simulink model "Magnetorquer"  (R2023b)
settings: Solver=FixedStepAuto  StartTime=0.0  StopTime=30  FixedStep=0.005  MaxStep=0.05  RelTol=1e-3
model workspace (MAT data in the model file):
  A = Simulink.Parameter
  A.Value = 0.00020106192
  A.DataType = 'auto'
  A.Complexity = 'real'
  A.Dimensions = [1 1]
  L = Simulink.Parameter
  L.Value = 0.1
  L.DataType = 'auto'
  L.Complexity = 'real'
  L.Dimensions = [1 1]
  M_s = Simulink.Parameter
  M_s.Value = 1600000
  M_s.DataType = 'auto'
  M_s.Complexity = 'real'
  M_s.Dimensions = [1 1]
  R = Simulink.Parameter
  R.Value = 4.0416
  R.DataType = 'auto'
  R.Complexity = 'real'
  R.Dimensions = [1 1]
  Sig = Simulink.Signal
  Sig.DataType = 'auto'
  Sig.Dimensions = -1
  Sig.DimensionsMode = 'auto'
  Sig.Complexity = 'auto'
  Sig.SampleTime = -1
  Sig.SamplingMode = 'auto'
  a = Simulink.Parameter
  a.Value = 1100
  a.DataType = 'auto'
  a.Complexity = 'real'
  a.Dimensions = [1 1]
  alpha = Simulink.Parameter
  alpha.Value = 0.0016
  alpha.DataType = 'auto'
  alpha.Complexity = 'real'
  alpha.Dimensions = [1 1]
  c = Simulink.Parameter
  c.Value = 0.2
  c.DataType = 'auto'
  c.Complexity = 'real'
  c.Dimensions = [1 1]
  k = Simulink.Parameter
  k.Value = 400
  k.DataType = 'auto'
  k.Complexity = 'real'
  k.Dimensions = [1 1]
  mu_0 = Simulink.Parameter
  mu_0.Value = 1.25663706212e-06
  mu_0.DataType = 'auto'
  mu_0.Complexity = 'real'
  mu_0.Dimensions = [1 1]
  n = Simulink.Parameter
  n.Value = 1000
  n.DataType = 'auto'
  n.Complexity = 'real'
  n.Dimensions = [1 1]
values from neighbouring files (symbols this model uses):
  a = 15    [quaternionTest.m]
  R = [1 - 2*(qj^2 + qk^2),  2*(qi*qj - qk*qr),   2*(qi*qk + qj*qr) ... (first row only)    [quat2rotmat.m]
settings Model: SnapshotBufferSize=20  SnapshotInterval=1  Creator=andrea  LastModifiedBy=andrea
settings SolverCC: ZeroCrossAlgorithm=Adaptive  SolverResetMethod=Robust
settings HardwareCC: ProdBitPerLong=64  ProdHWDeviceType=Intel->x86-64 (Linux 64)

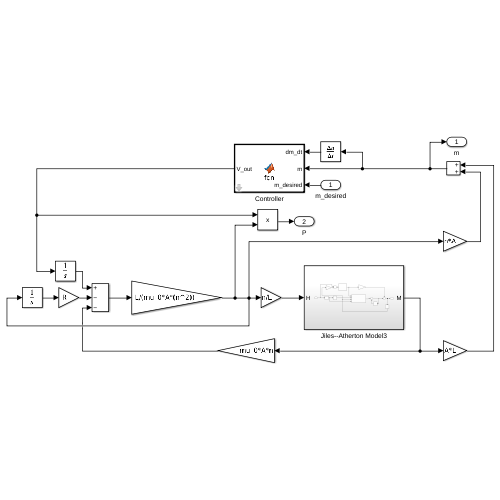
[thumbnail: Simulink's stored preview of the top-level diagram]
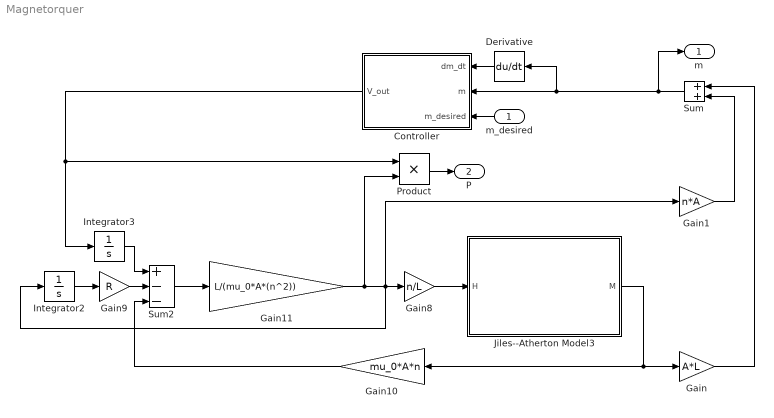
== system Magnetorquer ==
  m_desired : Inport
  Controller : MATLAB Function  TreatAsAtomicUnit=on  SystemSampleTime=0.005  mask{V=3.3, dt=0.005, e=0.5}
  Derivative : Derivative
  Gain : Gain  Gain=A*L
  Gain1 : Gain  Gain=n*A
  Gain10 : Gain  Gain=mu_0*A*n
  Gain11 : Gain  Gain=L/(mu_0*A*(n^2))
  Gain8 : Gain  Gain=n/L
  Gain9 : Gain  Gain=R
  Integrator2 : Integrator
  Integrator3 : Integrator
  Jiles--Atherton Model3 : Subsystem
  Product : Product
  Sum : Sum
  Sum2 : Sum  Inputs=+--
  m : Outport
  P : Outport  Port=2
  wires:
  Gain8/1 -> Jiles--Atherton Model3/1(H)
  Integrator2/1 -> Gain9/1
  Gain9/1 -> Sum2/2
  Integrator3/1 -> Sum2/1
  Sum2/1 -> Gain11/1
  Gain1/1 -> Sum/2
  Gain/1 -> Sum/1
  Sum/1 -> m/1, Derivative/1, Controller/2(m)
  Derivative/1 -> Controller/1(dm_dt)
  Gain11/1 -> Product/2, Gain1/1, Integrator2/1, Gain8/1
  Gain10/1 -> Sum2/3
  Jiles--Atherton Model3/1(M) -> Gain/1, Gain10/1
  Controller/1(V_out) -> Integrator3/1, Product/1
  m_desired/1 -> Controller/3(m_desired)
  Product/1 -> P/1

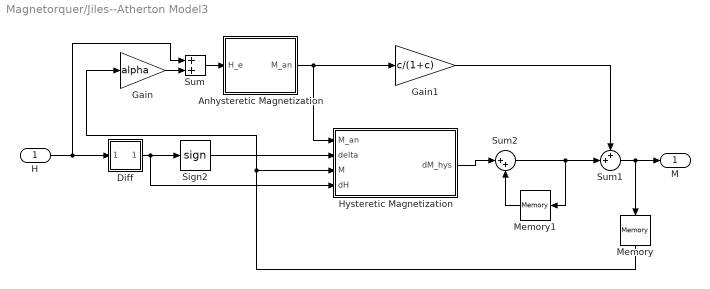
== system Magnetorquer/Jiles--Atherton Model3 ==
  H : Inport
  Anhysteretic Magnetization : MATLAB Function  TreatAsAtomicUnit=on  mask{M_s=M_s, a=a}
  Diff : Subsystem
  Gain : Gain  Gain=alpha
  Gain1 : Gain  Gain=c/(1+c)
  Hysteretic Magnetization : MATLAB Function  TreatAsAtomicUnit=on  mask{c=c, alpha=alpha, k=k}
  Memory : Memory
  Memory1 : Memory
  Sign2 : Signum
  Sum : Sum
  Sum1 : Sum  Inputs=++|
  Sum2 : Sum  Inputs=|++
  M : Outport
  wires:
  H/1 -> Sum/1, Diff/1(In1)
  Diff/1(Out1) -> Hysteretic Magnetization/4(dH), Sign2/1
  Sign2/1 -> Hysteretic Magnetization/2(delta)
  Gain/1 -> Sum/2
  Sum/1 -> Anhysteretic Magnetization/1(H_e)
  Memory/1 -> Hysteretic Magnetization/3(M), Gain/1
  Anhysteretic Magnetization/1(M_an) -> Gain1/1, Hysteretic Magnetization/1(M_an)
  Sum1/1 -> Memory/1, M/1
  Sum2/1 -> Memory1/1, Sum1/2
  Memory1/1 -> Sum2/2
  Hysteretic Magnetization/1(dM_hys) -> Sum2/1
  Gain1/1 -> Sum1/1

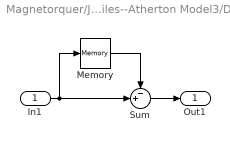
== system Magnetorquer/Jiles--Atherton Model3/Diff ==
  In1 : Inport
  Memory : Memory
  Sum : Sum  Inputs=-+|
  Out1 : Outport
  wires:
  In1/1 -> Memory/1, Sum/2
  Memory/1 -> Sum/1
  Sum/1 -> Out1/1

== matlab function Magnetorquer/Controller ==
  data: V_out output; dm_dt input; m input; m_desired input; V parameter; e parameter; dt parameter
function V_out = fcn(dm_dt, m, m_desired, V, e, dt)

if abs(m_desired-m) < e
    V_out = 0;
elseif abs((m_desired + dm_dt*dt)-m) < e
    V_out = 0;
else
    V_out = V*sign(m_desired-m);
end

== matlab function Magnetorquer/Jiles--Atherton Model3/Anhysteretic Magnetization ==
  data: H_e input; M_an output; M_s parameter; a parameter
function M_an = fcn(H_e, M_s, a)

if abs(H_e/a) <= 1e-5
    M_an = (1/3)*H_e/a;
else
    M_an = M_s * (coth(H_e/a)-a/H_e);
end

%H_e
%M_an

== matlab function Magnetorquer/Jiles--Atherton Model3/Hysteretic Magnetization ==
  data: M_an input; delta input; M input; dH input; dM_hys output; c parameter; k parameter; alpha parameter
function dM_hys = fcn(M_an, delta, M, dH, c, k, alpha)

if (M_an-M>0) && (delta<0)
    delta_m = 0;
elseif (M_an-M<0) && (delta>0)
    delta_m = 0;
else
    delta_m = 1;
end

if delta == 0
    delta = 1;
end

%dH
%dM_an
%delta
%M
%alpha
%thing1=(delta_m/(1+c))
%thing2=((M_an-M)/(delta*k-alpha*(M_an-M)))
%thing3=(M_an-M)
%thing4=(delta*k-alpha*(M_an-M))
%delta
dM_hys = (delta_m/(1+c))*((M_an-M)/(delta*k-alpha*(M_an-M)))*dH;
